simulink model "xieboduoji_13fangzhennow"  (R2023a)
settings: Solver=ode4  StartTime=0.0  StopTime=2.2  FixedStep=5e-7  RelTol=1e-3
undefined symbols (not defined in the file or in its folder): magnitude
libraries: simulink x417, spsRMSLib x70, spsCurrentMeasurementLib x32, spsVoltageMeasurementLib x31, powerlib_meascontrol x24, spsFourierLib x21, spsGroundLib x19, spsThreePhasePISectionLineLib x17, spsThreePhaseSeriesRLCBranchLib x14, spsdq0toAlphaBetaZeroLib x13, spsSeriesRLCBranchLib x11, spsUniversalBridgeLib x11
(part 11 of 12)

== system xieboduoji_13fangzhennow/node3/PV15kW3/谐波检测/Subsystem/Sub5 ==
  In1 : Inport
  Add : Sum
  Constant1 : Constant  Value=10*pi/180
  Constant{10,12,15,17} (4 alike) : Constant  Value=100*pi
  Constant11 : Constant  Value=19
  Constant2 : Constant  Value=10*pi/180
  Cos : Trigonometry  Operator=cos
  Cos1 : Trigonometry  Operator=cos
  Cos2 : Trigonometry
  Cos3 : Trigonometry
  Delay : Delay  DelayLength=400  SampleTime=5e-5
  Delay1 : Delay  DelayLength=1  SampleTime=5e-5
  Delay2 : Delay  DelayLength=1  SampleTime=5e-5
  Discrete PID Controller : slpidlib/PID Controller  Controller=P  Form=Parallel  TimeDomain=Discrete-time  UseExternalTs=off  SampleTime=5e-5  IntegratorMethod=Forward Euler  FilterMethod=Forward Euler  ControllerParametersSource=internal  P=1  I=1  UseKiTs=off  D=0  N=100  UseFilter=on  TunerSelectOption=Transfer Function Based (PID Tuner App)  InitialConditionSource=internal  InitialConditionForIntegrator=0  InitialConditionForFilter=0  DifferentiatorICPrevScaledInput=0  ExternalReset=none  TrackingMode=off  Kt=1  LimitOutput=off  SatLimitsSource=internal  UpperSaturationLimit=inf  LowerSaturationLimit=-inf  LinearizeAsGain=off  AntiWindupMode=none  Kb=1  LimitIntegrator=off  UpperIntegratorSaturationLimit=inf  LowerIntegratorSaturationLimit=-inf  POutMin=[]  POutMax=[]  IOutMin=[]  IOutMax=[]  DOutMin=[]  DOutMax=[]  NOutMin=[]  NOutMax=[]  SumOutMin=[]  SumOutMax=[]  SaturationOutMin=[]  SaturationOutMax=[]  PParamMin=[]  PParamMax=[]  IParamMin=[]  IParamMax=[]  DParamMin=[]  DParamMax=[]  NParamMin=[]  NParamMax=[]  KbParamMin=[]  KbParamMax=[]  KtParamMin=[]  KtParamMax=[]  KbOutMin=[]  KbOutMax=[]  KtOutMin=[]  KtOutMax=[]  IntegratorOutMin=[]  IntegratorOutMax=[]  FilterOutMin=[]  FilterOutMax=[]  SumI1OutMin=[]  SumI1OutMax=[]  SumI2OutMin=[]  SumI2OutMax=[]  SumI3OutMin=[]  SumI3OutMax=[]  SumI4OutMin=[]  SumI4OutMax=[]  SumDOutMin=[]  SumDOutMax=[]  DifferentiatorOutMin=[]  DifferentiatorOutMax=[]  FilterDiffOutCoefMin=[]  FilterDiffOutCoefMax=[]  ReciprocalOutMin=[]  ReciprocalOutMax=[]  SumDenOutMin=[]  SumDenOutMax=[]  SumNumOutMin=[]  SumNumOutMax=[]  DivideOutMin=[]  DivideOutMax=[]  UdiffTsProdOutMin=[]  UdiffTsProdOutMax=[]  NTsProdOutMin=[]  NTsProdOutMax=[]  UintegralTsProdOutMin=[]  UintegralTsProdOutMax=[]  UngainTsProdOutMin=[]  UngainTsProdOutMax=[]  ClampingZeroOutDataTypeStr=Inherit: Inherit via back propagation  ClampingZeroOutMin=[]  ClampingZeroOutMax=[]  FilterDenConstantOutDataTypeStr=Inherit: Inherit via back propagation  FilterDenConstantOutMin=[]  FilterDenConstantOutMax=[]  PCopyOutDataTypeStr=Inherit: Inherit via back propagation  PCopyOutMin=[]  PCopyOutMax=[]  NCopyOutDataTypeStr=Inherit: Inherit via back propagation  NCopyOutMin=[]  NCopyOutMax=[]  IntegratorContinuousStateAttributes=''  IntegratorStateMustResolveToSignalObject=off  IntegratorRTWStateStorageClass=Auto  FilterContinuousStateAttributes=''  FilterStateMustResolveToSignalObject=off  FilterRTWStateStorageClass=Auto  ParallelPVariant=InternalParameters  IdealPVariant=Disabled  IVariant=Disabled  DVariant=Disabled  IntegratorVariant=Disabled  SatVariant=Disabled  AWVariant=Disabled  PCopyVariant=Disabled  TRVariant=Disabled  FdbkBlocksVariant=Forward  IdealPFdbkVariant=Disabled  SatFdbkVariant=Disabled  DerivativeFilterVariant=Disabled  NVariant=Disabled  NCopyVariant=Disabled_SignalSpec  FilterICVariant=Disabled  IntegratorICVariant=Disabled  ExternalResetVariant=Disabled  TRSumVariant=Passthrough  SumFdbkVariant=Disabled  SumVariant=Passthrough_P  TsampFilterVariant=InternalTs  TsampNgainVariant=Passthrough  TsampIntegralVariant=Disabled_SignalSpec  ExternalSaturationOutDataTypeStr=Inherit: Same as second input
  Discrete PID Controller1 : slpidlib/PID Controller  Controller=P  Form=Parallel  TimeDomain=Discrete-time  UseExternalTs=off  SampleTime=5e-5  IntegratorMethod=Forward Euler  FilterMethod=Forward Euler  ControllerParametersSource=internal  P=1  I=1  UseKiTs=off  D=0  N=100  UseFilter=on  TunerSelectOption=Transfer Function Based (PID Tuner App)  InitialConditionSource=internal  InitialConditionForIntegrator=0  InitialConditionForFilter=0  DifferentiatorICPrevScaledInput=0  ExternalReset=none  TrackingMode=off  Kt=1  LimitOutput=off  SatLimitsSource=internal  UpperSaturationLimit=inf  LowerSaturationLimit=-inf  LinearizeAsGain=off  AntiWindupMode=none  Kb=1  LimitIntegrator=off  UpperIntegratorSaturationLimit=inf  LowerIntegratorSaturationLimit=-inf  POutMin=[]  POutMax=[]  IOutMin=[]  IOutMax=[]  DOutMin=[]  DOutMax=[]  NOutMin=[]  NOutMax=[]  SumOutMin=[]  SumOutMax=[]  SaturationOutMin=[]  SaturationOutMax=[]  PParamMin=[]  PParamMax=[]  IParamMin=[]  IParamMax=[]  DParamMin=[]  DParamMax=[]  NParamMin=[]  NParamMax=[]  KbParamMin=[]  KbParamMax=[]  KtParamMin=[]  KtParamMax=[]  KbOutMin=[]  KbOutMax=[]  KtOutMin=[]  KtOutMax=[]  IntegratorOutMin=[]  IntegratorOutMax=[]  FilterOutMin=[]  FilterOutMax=[]  SumI1OutMin=[]  SumI1OutMax=[]  SumI2OutMin=[]  SumI2OutMax=[]  SumI3OutMin=[]  SumI3OutMax=[]  SumI4OutMin=[]  SumI4OutMax=[]  SumDOutMin=[]  SumDOutMax=[]  DifferentiatorOutMin=[]  DifferentiatorOutMax=[]  FilterDiffOutCoefMin=[]  FilterDiffOutCoefMax=[]  ReciprocalOutMin=[]  ReciprocalOutMax=[]  SumDenOutMin=[]  SumDenOutMax=[]  SumNumOutMin=[]  SumNumOutMax=[]  DivideOutMin=[]  DivideOutMax=[]  UdiffTsProdOutMin=[]  UdiffTsProdOutMax=[]  NTsProdOutMin=[]  NTsProdOutMax=[]  UintegralTsProdOutMin=[]  UintegralTsProdOutMax=[]  UngainTsProdOutMin=[]  UngainTsProdOutMax=[]  ClampingZeroOutDataTypeStr=Inherit: Inherit via back propagation  ClampingZeroOutMin=[]  ClampingZeroOutMax=[]  FilterDenConstantOutDataTypeStr=Inherit: Inherit via back propagation  FilterDenConstantOutMin=[]  FilterDenConstantOutMax=[]  PCopyOutDataTypeStr=Inherit: Inherit via back propagation  PCopyOutMin=[]  PCopyOutMax=[]  NCopyOutDataTypeStr=Inherit: Inherit via back propagation  NCopyOutMin=[]  NCopyOutMax=[]  IntegratorContinuousStateAttributes=''  IntegratorStateMustResolveToSignalObject=off  IntegratorRTWStateStorageClass=Auto  FilterContinuousStateAttributes=''  FilterStateMustResolveToSignalObject=off  FilterRTWStateStorageClass=Auto  ParallelPVariant=InternalParameters  IdealPVariant=Disabled  IVariant=Disabled  DVariant=Disabled  IntegratorVariant=Disabled  SatVariant=Disabled  AWVariant=Disabled  PCopyVariant=Disabled  TRVariant=Disabled  FdbkBlocksVariant=Forward  IdealPFdbkVariant=Disabled  SatFdbkVariant=Disabled  DerivativeFilterVariant=Disabled  NVariant=Disabled  NCopyVariant=Disabled_SignalSpec  FilterICVariant=Disabled  IntegratorICVariant=Disabled  ExternalResetVariant=Disabled  TRSumVariant=Passthrough  SumFdbkVariant=Disabled  SumVariant=Passthrough_P  TsampFilterVariant=InternalTs  TsampNgainVariant=Passthrough  TsampIntegralVariant=Disabled_SignalSpec  ExternalSaturationOutDataTypeStr=Inherit: Same as second input
  Divide{,1..3} (4 alike) : Product  Inputs=***
  Dot Product{,1..5} (6 alike) : DotProduct  OutDataTypeStr=Inherit: Inherit via internal rule
  Gain : Gain  Gain=2/400
  Gain10 : Gain  Gain=2/400
  Ramp{,1..3} (4 alike) : simulink/Sources/Ramp  slope=1  start=0  InitialOutput=0
  Sqrt : Sqrt
  Sum{,1,3,9,18} (5 alike) : Sum  Inputs=|++
  Sum2 : Sum  Inputs=-+|
  u11 : Outport
  Out2 : Outport  Port=2
  wires:
  Constant17/1 -> Divide3/2
  Ramp/1 -> Divide/3
  Sum2/1 -> Dot Product2/1, Dot Product/2
  Divide/1 -> Cos/1
  Cos/1 -> Dot Product/1
  Dot Product/1 -> Gain/1
  Cos1/1 -> Dot Product1/1
  In1/1 -> Delay/1, Sum2/2
  Constant15/1 -> Divide2/2
  Sum18/1 -> Dot Product4/1, Discrete PID Controller1/1, Delay2/1
  [thk] -> Divide3/1
  [thk] -> Divide2/1
  Dot Product4/1 -> Sum9/2
  [thk] -> Divide1/1
  Ramp3/1 -> Divide3/3
  Delay1/1 -> Sum3/2
  Cos2/1 -> Dot Product2/2
  Dot Product2/1 -> Gain10/1
  Cos3/1 -> Dot Product4/2
  Divide2/1 -> Cos2/1
  Constant12/1 -> Divide1/2
  Ramp1/1 -> Divide1/3
  Delay/1 -> Sum2/1
  Sum3/1 -> Discrete PID Controller/1, Dot Product1/2, Delay1/1
  Gain10/1 -> Sum18/1
  Delay2/1 -> Sum18/2
  Constant10/1 -> Divide/2
  Ramp2/1 -> Divide2/3
  Gain/1 -> Sum3/1
  Dot Product1/1 -> Sum9/1
  Sum9/1 -> u11/1
  Constant11/1 -> [thk]
  [thk] -> Divide/1
  Dot Product3/1 -> Add/1
  Dot Product5/1 -> Add/2
  Add/1 -> Sqrt/1
  Sqrt/1 -> Out2/1
  Discrete PID Controller/1 -> Dot Product3/1, Dot Product3/2
  Discrete PID Controller1/1 -> Dot Product5/2, Dot Product5/1
  Divide1/1 -> Sum/1
  Sum/1 -> Cos1/1
  Divide3/1 -> Sum1/1
  Sum1/1 -> Cos3/1
  Constant1/1 -> Sum/2
  Constant2/1 -> Sum1/2

== system xieboduoji_13fangzhennow/node3/PV15kW3/谐波检测/Subsystem/Sub6 ==
  In1 : Inport
  Constant1 : Constant  Value=-60*pi/180
  Constant{10,12,15,17} (4 alike) : Constant  Value=100*pi
  Constant11 : Constant  Value=5
  Constant2 : Constant  Value=-60*pi/180
  Cos : Trigonometry  Operator=cos
  Cos1 : Trigonometry  Operator=cos
  Cos2 : Trigonometry
  Cos3 : Trigonometry
  Delay : Delay  DelayLength=400  SampleTime=5e-5
  Delay1 : Delay  DelayLength=1  SampleTime=5e-5
  Delay2 : Delay  DelayLength=1  SampleTime=5e-5
  Divide{,1..3} (4 alike) : Product  Inputs=***
  Dot Product{,1..2,4} (4 alike) : DotProduct  OutDataTypeStr=Inherit: Inherit via internal rule
  Gain : Gain  Gain=2/400
  Gain10 : Gain  Gain=2/400
  Ramp{,1..3} (4 alike) : simulink/Sources/Ramp  slope=1  start=0  InitialOutput=0
  Sum{,1,3,9,18} (5 alike) : Sum  Inputs=|++
  Sum2 : Sum  Inputs=-+|
  u1 : Outport
  wires:
  [thk] -> Divide/1
  Constant11/1 -> [thk]
  Sum9/1 -> u1/1
  Dot Product1/1 -> Sum9/1
  Gain/1 -> Sum3/1
  Ramp2/1 -> Divide2/3
  Constant10/1 -> Divide/2
  Delay2/1 -> Sum18/2
  Gain10/1 -> Sum18/1
  Sum3/1 -> Delay1/1, Dot Product1/2
  Delay/1 -> Sum2/1
  Ramp1/1 -> Divide1/3
  Constant12/1 -> Divide1/2
  Divide2/1 -> Cos2/1
  Cos3/1 -> Dot Product4/2
  Dot Product2/1 -> Gain10/1
  Cos2/1 -> Dot Product2/2
  Delay1/1 -> Sum3/2
  Ramp3/1 -> Divide3/3
  [thk] -> Divide1/1
  Dot Product4/1 -> Sum9/2
  [thk] -> Divide2/1
  [thk] -> Divide3/1
  Sum18/1 -> Delay2/1, Dot Product4/1
  Constant15/1 -> Divide2/2
  In1/1 -> Sum2/2, Delay/1
  Dot Product/1 -> Gain/1
  Cos/1 -> Dot Product/1
  Divide/1 -> Cos/1
  Sum2/1 -> Dot Product/2, Dot Product2/1
  Ramp/1 -> Divide/3
  Constant17/1 -> Divide3/2
  Cos1/1 -> Dot Product1/1
  Divide1/1 -> Sum/1
  Sum/1 -> Cos1/1
  Sum1/1 -> Cos3/1
  Divide3/1 -> Sum1/1

== system xieboduoji_13fangzhennow/node3/PV15kW3/谐波检测/Subsystem/Sub7 ==
  In1 : Inport
  Constant1 : Constant  Value=-60*pi/180
  Constant{10,12,15,17} (4 alike) : Constant  Value=100*pi
  Constant11 : Constant  Value=7
  Constant2 : Constant  Value=-60*pi/180
  Cos : Trigonometry  Operator=cos
  Cos1 : Trigonometry  Operator=cos
  Cos2 : Trigonometry
  Cos3 : Trigonometry
  Delay : Delay  DelayLength=400  SampleTime=5e-5
  Delay1 : Delay  DelayLength=1  SampleTime=5e-5
  Delay2 : Delay  DelayLength=1  SampleTime=5e-5
  Divide{,1..3} (4 alike) : Product  Inputs=***
  Dot Product{,1..2,4} (4 alike) : DotProduct  OutDataTypeStr=Inherit: Inherit via internal rule
  Gain : Gain  Gain=2/400
  Gain10 : Gain  Gain=2/400
  Ramp{,1..3} (4 alike) : simulink/Sources/Ramp  slope=1  start=0  InitialOutput=0
  Sum{,1,3,9,18} (5 alike) : Sum  Inputs=|++
  Sum2 : Sum  Inputs=-+|
  u1 : Outport
  wires:
  Divide3/1 -> Sum1/1
  Sum1/1 -> Cos3/1
  Sum/1 -> Cos1/1
  Divide1/1 -> Sum/1
  Cos1/1 -> Dot Product1/1
  Constant17/1 -> Divide3/2
  Ramp/1 -> Divide/3
  Sum2/1 -> Dot Product2/1, Dot Product/2
  Divide/1 -> Cos/1
  Cos/1 -> Dot Product/1
  Dot Product/1 -> Gain/1
  In1/1 -> Delay/1, Sum2/2
  Constant15/1 -> Divide2/2
  Sum18/1 -> Dot Product4/1, Delay2/1
  [thk] -> Divide3/1
  [thk] -> Divide2/1
  Dot Product4/1 -> Sum9/2
  [thk] -> Divide1/1
  Ramp3/1 -> Divide3/3
  Delay1/1 -> Sum3/2
  Cos2/1 -> Dot Product2/2
  Dot Product2/1 -> Gain10/1
  Cos3/1 -> Dot Product4/2
  Divide2/1 -> Cos2/1
  Constant12/1 -> Divide1/2
  Ramp1/1 -> Divide1/3
  Delay/1 -> Sum2/1
  Sum3/1 -> Dot Product1/2, Delay1/1
  Gain10/1 -> Sum18/1
  Delay2/1 -> Sum18/2
  Constant10/1 -> Divide/2
  Ramp2/1 -> Divide2/3
  Gain/1 -> Sum3/1
  Dot Product1/1 -> Sum9/1
  Sum9/1 -> u1/1
  Constant11/1 -> [thk]
  [thk] -> Divide/1

== system xieboduoji_13fangzhennow/node3/PV15kW3/谐波检测/Subsystem/Sub8 ==
  In1 : Inport
  Constant1 : Constant  Value=-15*pi/180
  Constant{10,12,15,17} (4 alike) : Constant  Value=100*pi
  Constant11 : Constant  Value=11
  Constant2 : Constant  Value=-15*pi/180
  Cos : Trigonometry  Operator=cos
  Cos2 : Trigonometry
  Cos3 : Trigonometry
  Cos4 : Trigonometry  Operator=cos
  Delay : Delay  DelayLength=400  SampleTime=5e-5
  Delay1 : Delay  DelayLength=1  SampleTime=5e-5
  Delay2 : Delay  DelayLength=1  SampleTime=5e-5
  Divide{,1..3} (4 alike) : Product  Inputs=***
  Dot Product{,1..2,4} (4 alike) : DotProduct  OutDataTypeStr=Inherit: Inherit via internal rule
  Gain : Gain  Gain=2/400
  Gain10 : Gain  Gain=2/400
  Ramp{,1..3} (4 alike) : simulink/Sources/Ramp  slope=1  start=0  InitialOutput=0
  Sum{,1,3,9,18} (5 alike) : Sum  Inputs=|++
  Sum2 : Sum  Inputs=-+|
  u5 : Outport
  wires:
  Sum1/1 -> Cos3/1
  Constant1/1 -> Sum1/2
  Divide3/1 -> Sum1/1
  Cos4/1 -> Dot Product1/1
  Sum/1 -> Cos4/1
  Constant2/1 -> Sum/2
  Divide1/1 -> Sum/1
  Constant17/1 -> Divide3/2
  Ramp/1 -> Divide/3
  Sum2/1 -> Dot Product2/1, Dot Product/2
  Divide/1 -> Cos/1
  Cos/1 -> Dot Product/1
  Dot Product/1 -> Gain/1
  In1/1 -> Delay/1, Sum2/2
  Constant15/1 -> Divide2/2
  Sum18/1 -> Dot Product4/1, Delay2/1
  [thk] -> Divide3/1
  [thk] -> Divide2/1
  Dot Product4/1 -> Sum9/2
  [thk] -> Divide1/1
  Ramp3/1 -> Divide3/3
  Delay1/1 -> Sum3/2
  Cos2/1 -> Dot Product2/2
  Dot Product2/1 -> Gain10/1
  Cos3/1 -> Dot Product4/2
  Divide2/1 -> Cos2/1
  Constant12/1 -> Divide1/2
  Ramp1/1 -> Divide1/3
  Delay/1 -> Sum2/1
  Sum3/1 -> Dot Product1/2, Delay1/1
  Gain10/1 -> Sum18/1
  Delay2/1 -> Sum18/2
  Constant10/1 -> Divide/2
  Ramp2/1 -> Divide2/3
  Gain/1 -> Sum3/1
  Dot Product1/1 -> Sum9/1
  Sum9/1 -> u5/1
  Constant11/1 -> [thk]
  [thk] -> Divide/1

== system xieboduoji_13fangzhennow/node3/PV15kW3/谐波检测/Subsystem/Sub9 ==
  In1 : Inport
  Constant1 : Constant  Value=-15*pi/180
  Constant{10,12,15,17} (4 alike) : Constant  Value=100*pi
  Constant11 : Constant  Value=13
  Constant2 : Constant  Value=-15*pi/180
  Cos : Trigonometry  Operator=cos
  Cos1 : Trigonometry  Operator=cos
  Cos2 : Trigonometry
  Cos3 : Trigonometry
  Delay : Delay  DelayLength=400  SampleTime=5e-5
  Delay1 : Delay  DelayLength=1  SampleTime=5e-5
  Delay2 : Delay  DelayLength=1  SampleTime=5e-5
  Divide{,1..3} (4 alike) : Product  Inputs=***
  Dot Product{,1..2,4} (4 alike) : DotProduct  OutDataTypeStr=Inherit: Inherit via internal rule
  Gain : Gain  Gain=2/400
  Gain10 : Gain  Gain=2/400
  Ramp{,1..3} (4 alike) : simulink/Sources/Ramp  slope=1  start=0  InitialOutput=0
  Sum{,1,3,9,18} (5 alike) : Sum  Inputs=|++
  Sum2 : Sum  Inputs=-+|
  u7 : Outport
  wires:
  Sum1/1 -> Cos3/1
  Constant1/1 -> Sum1/2
  Divide3/1 -> Sum1/1
  Sum/1 -> Cos1/1
  Constant2/1 -> Sum/2
  Divide1/1 -> Sum/1
  [thk] -> Divide/1
  Constant11/1 -> [thk]
  Sum9/1 -> u7/1
  Dot Product1/1 -> Sum9/1
  Gain/1 -> Sum3/1
  Ramp2/1 -> Divide2/3
  Constant10/1 -> Divide/2
  Delay2/1 -> Sum18/2
  Gain10/1 -> Sum18/1
  Sum3/1 -> Delay1/1, Dot Product1/2
  Delay/1 -> Sum2/1
  Ramp1/1 -> Divide1/3
  Constant12/1 -> Divide1/2
  Divide2/1 -> Cos2/1
  Cos3/1 -> Dot Product4/2
  Dot Product2/1 -> Gain10/1
  Cos2/1 -> Dot Product2/2
  Delay1/1 -> Sum3/2
  Ramp3/1 -> Divide3/3
  [thk] -> Divide1/1
  Dot Product4/1 -> Sum9/2
  [thk] -> Divide2/1
  [thk] -> Divide3/1
  Sum18/1 -> Delay2/1, Dot Product4/1
  Constant15/1 -> Divide2/2
  In1/1 -> Sum2/2, Delay/1
  Cos1/1 -> Dot Product1/1
  Dot Product/1 -> Gain/1
  Cos/1 -> Dot Product/1
  Divide/1 -> Cos/1
  Sum2/1 -> Dot Product/2, Dot Product2/1
  Ramp/1 -> Divide/3
  Constant17/1 -> Divide3/2

== system xieboduoji_13fangzhennow/node3/PV15kW3/谐波检测/Subsystem/Subsystem2 ==
  u1 : Inport
  u2 : Inport  Port=2
  u3 : Inport  Port=3
  u4 : Inport  Port=4
  u5 : Inport  Port=5
  u6 : Inport  Port=6
  u7 : Inport  Port=7
  u8 : Inport  Port=8
  u9 : Inport  Port=9
  u10 : Inport  Port=10
  u11 : Inport  Port=11
  u12 : Inport  Port=12
  Pul : DiscretePulseGenerator  PulseType=Time based  Period=5e-5  PulseWidth=40
  RMS1 : Subsystem  TreatAsAtomicUnit=on
  k1 : Outport  VectorParamsAs1DForOutWhenUnconnected=off
  k2 : Outport  Port=2  VectorParamsAs1DForOutWhenUnconnected=off
  k3 : Outport  Port=3  VectorParamsAs1DForOutWhenUnconnected=off
  k4 : Outport  Port=4  VectorParamsAs1DForOutWhenUnconnected=off
  k5 : Outport  Port=5  VectorParamsAs1DForOutWhenUnconnected=off
  k6 : Outport  Port=6  VectorParamsAs1DForOutWhenUnconnected=off
  wires:
  Pul/1 -> RMS1/Trigger
  u1/1 -> RMS1/1(u1)
  u2/1 -> RMS1/2(i1)
  u3/1 -> RMS1/3(u3)
  u4/1 -> RMS1/4(u4)
  u5/1 -> RMS1/5(u5)
  u6/1 -> RMS1/6(u6)
  RMS1/2(k2) -> k2/1
  RMS1/3(k3) -> k3/1
  RMS1/4(k4) -> k4/1
  RMS1/1(k1) -> k1/1
  RMS1/6(k6) -> k6/1
  RMS1/5(k5) -> k5/1
  u12/1 -> RMS1/12(u10)
  u11/1 -> RMS1/11(u9)
  u10/1 -> RMS1/10(u8)
  u9/1 -> RMS1/9(u7)
  u8/1 -> RMS1/8(i2)
  u7/1 -> RMS1/7(u2)

== system xieboduoji_13fangzhennow/node3/PV15kW3/谐波检测/Subsystem2/RMS1 ==
  u1 : Inport
  i1 : Inport  Port=2
  u3 : Inport  Port=3
  u4 : Inport  Port=4
  u5 : Inport  Port=5
  u6 : Inport  Port=6
  u2 : Inport  Port=7
  i2 : Inport  Port=8
  u7 : Inport  Port=9
  u8 : Inport  Port=10
  u9 : Inport  Port=11
  u10 : Inport  Port=12
  Trigger : TriggerPort  VariantControl=(inherit)
  Scope : Scope
  xiebodianliu : MATLAB Function  Commented=on  TreatAsAtomicUnit=on
  xunidiandao : MATLAB Function  TreatAsAtomicUnit=on
  k1 : Outport  VectorParamsAs1DForOutWhenUnconnected=off
  k2 : Outport  Port=2  VectorParamsAs1DForOutWhenUnconnected=off
  k3 : Outport  Port=3  VectorParamsAs1DForOutWhenUnconnected=off
  k4 : Outport  Port=4  VectorParamsAs1DForOutWhenUnconnected=off
  k5 : Outport  Port=5  VectorParamsAs1DForOutWhenUnconnected=off
  k6 : Outport  Port=6  VectorParamsAs1DForOutWhenUnconnected=off
  wires:
  xunidiandao/1(k1) -> k1/1
  u1/1 -> xunidiandao/1(u1)
  xunidiandao/2(k2) -> k2/1
  xunidiandao/3(k3) -> k3/1
  xunidiandao/4(k4) -> k4/1
  xunidiandao/5(k5) -> k5/1
  xunidiandao/6(k6) -> k6/1
  i1/1 -> xunidiandao/2(i1)
  u3/1 -> xunidiandao/3(u2)
  u4/1 -> xunidiandao/4(i2)
  u5/1 -> xunidiandao/5(u3)
  u6/1 -> xunidiandao/6(i3)
  u10/1 -> xunidiandao/12(i6)
  u9/1 -> xunidiandao/11(u6)
  u8/1 -> xunidiandao/10(i5)
  u7/1 -> xunidiandao/9(u5)
  i2/1 -> xunidiandao/8(i4)
  u2/1 -> xunidiandao/7(u4)
  xunidiandao/7(k0) -> Scope/1

== system xieboduoji_13fangzhennow/node12/PV15kW3/谐波检测/Subsystem/Subsystem2/RMS1 ==
  u1 : Inport
  i1 : Inport  Port=2
  u3 : Inport  Port=3
  u4 : Inport  Port=4
  u5 : Inport  Port=5
  u6 : Inport  Port=6
  u2 : Inport  Port=7
  i2 : Inport  Port=8
  u7 : Inport  Port=9
  u8 : Inport  Port=10
  u9 : Inport  Port=11
  u10 : Inport  Port=12
  Trigger : TriggerPort  VariantControl=(inherit)
  Scope : Scope
  xiebodianliu : MATLAB Function  TreatAsAtomicUnit=on
  k1 : Outport  VectorParamsAs1DForOutWhenUnconnected=off
  k2 : Outport  Port=2  VectorParamsAs1DForOutWhenUnconnected=off
  k3 : Outport  Port=3  VectorParamsAs1DForOutWhenUnconnected=off
  k4 : Outport  Port=4  VectorParamsAs1DForOutWhenUnconnected=off
  k5 : Outport  Port=5  VectorParamsAs1DForOutWhenUnconnected=off
  k6 : Outport  Port=6  VectorParamsAs1DForOutWhenUnconnected=off
  wires:
  xiebodianliu/1(k1) -> k1/1
  u1/1 -> xiebodianliu/1(u1)
  xiebodianliu/2(k2) -> k2/1
  xiebodianliu/3(k3) -> k3/1
  xiebodianliu/4(k4) -> k4/1
  xiebodianliu/5(k5) -> k5/1
  xiebodianliu/6(k6) -> k6/1
  i1/1 -> xiebodianliu/2(i1)
  u3/1 -> xiebodianliu/3(u2)
  u4/1 -> xiebodianliu/4(i2)
  u5/1 -> xiebodianliu/5(u3)
  u6/1 -> xiebodianliu/6(i3)
  u10/1 -> xiebodianliu/12(i6)
  u9/1 -> xiebodianliu/11(u6)
  u8/1 -> xiebodianliu/10(i5)
  u7/1 -> xiebodianliu/9(u5)
  i2/1 -> xiebodianliu/8(i4)
  u2/1 -> xiebodianliu/7(u4)
  xiebodianliu/7(k0) -> Scope/1

== system xieboduoji_13fangzhennow/node3/PV15kW2/谐波检测/DFT6-24A1/Subsystem9/integral  ==
  di : Inport
  Trigger : TriggerPort  VariantControl=(inherit)
  Embedded MATLAB Function : MATLAB Function  TreatAsAtomicUnit=on
  w : Outport
  wires:
  Embedded MATLAB Function/1(w) -> w/1
  di/1 -> Embedded MATLAB Function/1(er)

== system xieboduoji_13fangzhennow/node3/PV15kW3/谐波检测/Subsystem/Subsystem2/RMS1 ==
  u1 : Inport
  i1 : Inport  Port=2
  u3 : Inport  Port=3
  u4 : Inport  Port=4
  u5 : Inport  Port=5
  u6 : Inport  Port=6
  u2 : Inport  Port=7
  i2 : Inport  Port=8
  u7 : Inport  Port=9
  u8 : Inport  Port=10
  u9 : Inport  Port=11
  u10 : Inport  Port=12
  Trigger : TriggerPort  VariantControl=(inherit)
  Scope : Scope
  xiebodianliu : MATLAB Function  TreatAsAtomicUnit=on
  xiebodianliu1 : MATLAB Function  Commented=on  TreatAsAtomicUnit=on
  k1 : Outport  VectorParamsAs1DForOutWhenUnconnected=off
  k2 : Outport  Port=2  VectorParamsAs1DForOutWhenUnconnected=off
  k3 : Outport  Port=3  VectorParamsAs1DForOutWhenUnconnected=off
  k4 : Outport  Port=4  VectorParamsAs1DForOutWhenUnconnected=off
  k5 : Outport  Port=5  VectorParamsAs1DForOutWhenUnconnected=off
  k6 : Outport  Port=6  VectorParamsAs1DForOutWhenUnconnected=off
  wires:
  xiebodianliu/1(k1) -> k1/1
  u1/1 -> xiebodianliu/1(u1)
  xiebodianliu/2(k2) -> k2/1
  xiebodianliu/3(k3) -> k3/1
  xiebodianliu/4(k4) -> k4/1
  xiebodianliu/5(k5) -> k5/1
  xiebodianliu/6(k6) -> k6/1
  i1/1 -> xiebodianliu/2(i1)
  u3/1 -> xiebodianliu/3(u2)
  u4/1 -> xiebodianliu/4(i2)
  u5/1 -> xiebodianliu/5(u3)
  u6/1 -> xiebodianliu/6(i3)
  u10/1 -> xiebodianliu/12(i6)
  u9/1 -> xiebodianliu/11(u6)
  u8/1 -> xiebodianliu/10(i5)
  u7/1 -> xiebodianliu/9(u5)
  i2/1 -> xiebodianliu/8(i4)
  u2/1 -> xiebodianliu/7(u4)
  xiebodianliu/7(k0) -> Scope/1

== matlab function xieboduoji_13fangzhennow/node3/Subsystem2/RMS1/xunidiandao ==
  data: y1 output; u1 input; u2 input; u3 input; u4 input; u5 input; u6 input; y11 output; y2 output; y22 output; y3 output; y33 output; y4 output; y44 output; y5 output; y55 output; y6 output; y66 output; x output
function [y1,y11,y2,y22,y3,y33,y4,y44,y5,y55,y6,y66,x] = Algorithm(u1,u2,u3,u4,u5,u6)

%控制器参数
T=5e-5;
persistent time;
persistent sum1 sum2 sum3 sum4 sum5 sum6;
persistent sum11 sum22 sum33 sum44 sum55 sum66;
persistent a1 a11 a2 a22 a3 a33 a4 a44 a5 a55 a6 a66
dataType = 'double';

%首次赋值
 if isempty(time)
time=20e-5;
sum1=0;sum2=0;sum3=0;sum4=0;sum5=0;sum6=0;
sum11=0;sum22=0;sum33=0;sum44=0;sum55=0;sum66=0;
a1=0;a11=0;a2=0;a22=0;a3=0;a33=0;a4=0;a44=0;a5=0;a55=0;a6=0;a66=0;
 end

 time=time+T;
  
 if (time>=0.9)&&(time<1.0)
     sum1=sum1+u1;sum2=sum2+u2;sum3=sum3+u3;
     sum4=sum4+u4;sum5=sum5+u5;sum6=sum6+u6;
 end
 if time>=1.0
     a1=sum1*0.0005;a2=sum2*0.0005;a3=sum3*0.0005;
     a4=sum4*0.0005;a5=sum5*0.0005;a6=sum6*0.0005;
 end
  if (time>=1.9)&&(time<2.0)
     sum11=sum11+u1;sum22=sum22+u2;sum33=sum33+u3;
     sum44=sum44+u4;sum55=sum55+u5;sum66=sum66+u6;
 end
 if time>=2.0
     a11=sum11*0.0005;a22=sum22*0.0005;a33=sum33*0.0005;
     a44=sum44*0.0005;a55=sum55*0.0005;a66=sum66*0.0005;
 end
 y1=a1;y2=a2;y3=a3;y4=a4;y5=a5;y6=a6;
 y11=a11;y22=a22;y33=a33;y44=a44;y55=a55;y66=a66;x=time+sum1;
end

== matlab function xieboduoji_13fangzhennow/node14/PV15kW3/谐波检测/Subsystem2/RMS1/xunidiandao ==
  data: k1 output; u1 input; i1 input; u2 input; i2 input; u3 input; i3 input; u4 input; i4 input; u5 input; i5 input; u6 input; k2 output; k3 output; k4 output; k5 output; k6 output; i6 input; k0 output
function [k1,k2,k3,k4,k5,k6,k0] = Algorithm(u1,i1,u2,i2,u3,i3,u4,i4,u5,i5,u6,i6)

%控制器参数
T=5e-5;
kp=0.01;
persistent low lim im k time;
persistent k11 k22 k33 k44 k55 k66 sumc;
persistent h1 flg1 sum1 out1 bao1 ki1;
persistent h2 flg2 sum2 out2 bao2 ki2;
persistent h3 flg3 sum3 out3 bao3 ki3;
persistent h4 flg4 sum4 out4 bao4 ki4;
persistent h5 flg5 sum5 out5 bao5 ki5;
persistent h6 flg6 sum6 out6 bao6 ki6;
dataType = 'double';

%首次赋值
 if isempty(k)
 low=311*0.25;lim=5;im=0;k=1;time=5e-5;%1.1
 k11=0;k22=0;k33=0;k44=0;k55=0;k66=0;sumc=0;
 h1=1;flg1=1;sum1=1;out1=1;bao1=0;ki1=25;
 h2=1;flg2=1;sum2=1;out2=1;bao2=0;ki2=25;
 h3=1;flg3=1;sum3=1;out3=1;bao3=0;ki3=25;
 h4=1;flg4=1;sum4=1;out4=1;bao4=0;ki4=25;
 h5=1;flg5=1;sum5=1;out5=1;bao5=0;ki5=25;
 h6=1;flg6=1;sum6=1;out6=1;bao6=0;ki6=25;
 end
   if (flg5==0)&&(flg6==0)
       sumc=sqrt((i5*out5)^2+(i6*out6)^2);
    if sumc>lim
        k11=k11*lim/sumc;out1=k11;sum1=k11;
        k22=k22*lim/sumc;out2=k22;sum2=k22;
        k33=k33*lim/sumc;out3=k33;sum3=k33;
        k44=k44*lim/sumc;out4=k44;sum4=k44;
        k55=k55*lim/sumc;out5=k55;sum5=k55;
        k66=k66*lim/sumc;out6=k66;sum6=k66;end 
   end
    if flg1==1
      h1=1;
    else h1=out1/k;end
    if flg2==1
      h2=1;
    else h2=out2/k;end
    if flg3==1
      h3=1;
    else h3=out3/k;end   
    if flg4==1
      h4=1;
    else h4=out4/k;end   
    if flg5==1
      h5=1;
    else h5=out5/k;end 
    if flg6==1
      h6=1;
    else h6=out6/k;end   
 im=sqrt((i1*h1)^2+(i2*h2)^2+(i3*h3)^2+(i4*h4)^2+(i5*h5)^2+(i6*h6)^2);%
 time=time+T;  
 k=lim/im;
     if k>3
     k=3;end
     if flg1==1
     k11=k;end
     if flg2==1
     k22=k;end 
     if flg3==1
     k33=k;end
     if flg4==1
     k44=k;end
     if flg5==1
     k55=k;end
     if flg6==1
     k66=k;end
  
 if time<1
     k11=0;k22=0;k33=0;k44=0;k55=0;k66=0;
 end
 if time>=1
     % if time>=1.4
     % low=1.02;end%1.02
     % if time>=1.7
     % low=0.512;end%0.512
  if time>=1.4
lim=10.6-time*4.0;lim1=10.6-time*4.0;
    if lim<4
    lim=4;lim1=4;
    end
  end
  
 er6=u6*1.414-low;er5=u5*1.414-low;
    if (er5<-0.06)||(er5>0.06)
         if (er5>0.06)%
         flg5=1;end
         if (er5<-0.06) 
          if flg5==1
          sum5=k;out5=k;end
         flg5=0;end   
    sum5=ki5*T*er5+sum5;out5=kp*er5+sum5;
        if flg5==0 
        k55=out5;end
     if(out5>k)
     flg5=1;out5=k;ki5=0;bao5=1;end
     if(out5<0)
     out5=0;ki5=0;bao5=1;end
     if(bao5==0)
     ki5=40;end
     bao5=0;
   end
    if (er6<-0.06)||(er6>0.06)
         if (er6>0.06)%
         flg6=1;end
         if (er6<-0.06) 
           if flg6==1
           sum6=k;out6=k;end
         flg6=0;end   
     sum6=ki6*T*er6+sum6; out6=kp*er6+sum6;
        if flg6==0 
        k66=out6;end
     if(out6>k)
     flg6=1;out6=k;ki6=0;bao6=1;end
     if(out6<0)
     out6=0;ki6=0;bao6=1;end
     if(bao6==0)
     ki6=40;end
     bao6=0;
    end
 end
 
 k1=k11;k2=k22;k3=k33;k4=k44;k5=k55;k6=k66;k0=flg6;
end

== matlab function xieboduoji_13fangzhennow/node12/PV15kW3/Subsystem9/integral /Embedded MATLAB Function ==
  data: er input; w output
function w  = Algorithm(er)

%控制器参数
Ts=10e-5;%控制周期，原始0.3-6
Kp=0.3;Ki0=8;n=35;
persistent n_sum dcbaohe Ki;
dataType = 'double';

%首次赋值
if isempty(n_sum)
    n_sum=0;dcbaohe=0;Ki=Ki0;
end
 
     n_sum=Ki*Ts*(er)+n_sum;
     outn=Kp*(er)+n_sum;
     if(outn>n)
     outn=n;Ki=0;dcbaohe=1;
     end
     if(outn<-n)
     outn=-n;Ki=0;dcbaohe=1;
     end
     if(dcbaohe==0)
         Ki=Ki0;
     end
     dcbaohe=0;
     
  w=outn; 
end

== matlab function xieboduoji_13fangzhennow/node12/PV15kW3/改进PLL1/PI/Embedded MATLAB Function ==
  data: Vgq input; w output
function w  = Algorithm(Vgq)

%控制器参数
T=5e-5;%控制周期

Kpllp=0.2;
Kplli=4;

persistent PLLsum;
persistent nsum2;

dataType = 'double';

%首次赋值
if isempty(PLLsum)
    PLLsum=0;
    nsum2=0;
end


w=Kpllp*Vgq+Kplli*(T*Vgq+PLLsum);
PLLsum=T*Vgq+PLLsum;
end

== matlab function xieboduoji_13fangzhennow/node3/PV15kW3/谐波检测/Subsystem/Subsystem2/RMS1/xiebodianliu ==
  data: k1 output; u1 input; i1 input; u2 input; i2 input; u3 input; i3 input; u4 input; i4 input; u5 input; i5 input; u6 input; k2 output; k3 output; k4 output; k5 output; k6 output; i6 input; k0 output
function [k1,k2,k3,k4,k5,k6,k0] = Algorithm(u1,i1,u2,i2,u3,i3,u4,i4,u5,i5,u6,i6)

%控制器参数
T=5e-5;
kp=0.01;
persistent lim lim1 im k time;
persistent k11 k22 k33 k44 k55 k66;
persistent flg1 flg2 flg3 flg4 flg5 flg6;
dataType = 'double';

%首次赋值
 if isempty(k)
 lim=5;lim1=5;im=0;k=1;time=5e-5;
 k11=0;k22=0;k33=0;k44=0;k55=0;k66=0;
 flg1=1; flg2=1; flg3=1; flg4=1; flg5=1; flg6=1;
 end
h1=1/0.6464;h2=1/0.7219;h3=1/1;
h4=1/0.9880;h5=1/0.5562;h6=1/0.6416;

im=sqrt(flg1*i1^2+flg2*i2^2+flg3*i3^2+flg4*i4^2+flg5*i5^2+flg6*i6^2);
it=(lim^2-((1-flg1)*h1*i1)^2-((1-flg2)*h2*i2)^2-((1-flg3)*h3*i3)^2-((1-flg4)*h4*i4)^2-((1-flg5)*h5*i5)^2-((1-flg6)*h6*i6)^2);
 if it>=0
 lim1=sqrt(it);
  if im>0
  k=lim1/im;end
 else
 lim1=0;k=0.7;
 end
time=time+T;
 if k>2
 k=2;end
     if k>h1
      k11=h1;flg1=0;
      else
      flg1=1;k11=k;end
     if k>h2
      k22=h2;flg2=0;
      else
      flg2=1;k22=k;end
     if k>h3
      k33=h3;flg3=0;
      else
      flg3=1;k33=k;end
     if k>h4
      k44=h4;flg4=0;
      else
      flg4=1;k44=k;end
     if k>h5
      k55=h5;flg5=0;
      else
      flg5=1;k55=k;end
     if k>h6
      k66=h6;flg6=0;
      else
      flg6=1;k66=k;end

  
 if time<1
     k11=0;k22=0;k33=0;k44=0;k55=0;k66=0;
 end
 if time>=1.4
lim=10.6-time*4.0;lim1=10.6-time*4.0;
    if lim<4
    lim=4;lim1=4;
    end
 end
 
 k1=k11;k2=k22;k3=k33;k4=k44;k5=k55;k6=k66;k0=it;
end

== matlab function xieboduoji_13fangzhennow/node12/PV15kW3/谐波检测/Subsystem/Subsystem2/RMS1/xiebodianliu ==
  data: k1 output; u1 input; i1 input; u2 input; i2 input; u3 input; i3 input; u4 input; i4 input; u5 input; i5 input; u6 input; k2 output; k3 output; k4 output; k5 output; k6 output; i6 input; k0 output
function [k1,k2,k3,k4,k5,k6,k0] = Algorithm(u1,i1,u2,i2,u3,i3,u4,i4,u5,i5,u6,i6)

%控制器参数
T=5e-5;
kp=0.01;
persistent lim lim1 im k time;
persistent k11 k22 k33 k44 k55 k66;
persistent flg1 flg2 flg3 flg4 flg5 flg6;
dataType = 'double';

%首次赋值
 if isempty(k)
 lim=5;lim1=5;im=0;k=1;time=5e-5;
 k11=0;k22=0;k33=0;k44=0;k55=0;k66=0;
 flg1=1; flg2=1; flg3=1; flg4=1; flg5=1; flg6=1;
 end
h1=1/0.7237;h2=1/0.8217;h3=1/1;
h4=1/1;h5=1/1;h6=1/1;

im=sqrt(flg1*i1^2+flg2*i2^2+flg3*i3^2+flg4*i4^2+flg5*i5^2+flg6*i6^2);
it=(lim^2-((1-flg1)*h1*i1)^2-((1-flg2)*h2*i2)^2-((1-flg3)*h3*i3)^2-((1-flg4)*h4*i4)^2-((1-flg5)*h5*i5)^2-((1-flg6)*h6*i6)^2);
 if it>=0
 lim1=sqrt(it);
  if im>0
  k=lim1/im;end
 else
 lim1=0;k=0.7;
 end
time=time+T;
 if k>2
 k=2;end
     if k>h1
      k11=h1;flg1=0;
      else
      flg1=1;k11=k;end
     if k>h2
      k22=h2;flg2=0;
      else
      flg2=1;k22=k;end
     if k>h3
      k33=h3;flg3=0;
      else
      flg3=1;k33=k;end
     if k>h4
      k44=h4;flg4=0;
      else
      flg4=1;k44=k;end
     if k>h5
      k55=h5;flg5=0;
      else
      flg5=1;k55=k;end
     if k>h6
      k66=h6;flg6=0;
      else
      flg6=1;k66=k;end

  
 if time<1
     k11=0;k22=0;k33=0;k44=0;k55=0;k66=0;
 end
 if time>=1.4
lim=10.6-time*4.0;lim1=10.6-time*4.0;
    if lim<4
    lim=4;lim1=4;
    end
 end
 
 k1=k11;k2=k22;k3=k33;k4=k44;k5=k55;k6=k66;k0=it;
end

== matlab function xieboduoji_13fangzhennow/node3/PV15kW3/Subsystem9/integral /Embedded MATLAB Function ==
  data: er input; w output
function w  = Algorithm(er)

%控制器参数
Ts=10e-5;%控制周期，原始0.3-6
Kp=0.3;Ki0=8;n=35;
persistent n_sum dcbaohe Ki;
dataType = 'double';

%首次赋值
if isempty(n_sum)
    n_sum=0;dcbaohe=0;Ki=Ki0;
end
 
     n_sum=Ki*Ts*(er)+n_sum;
     outn=Kp*(er)+n_sum;
     if(outn>n)
     outn=n;Ki=0;dcbaohe=1;
     end
     if(outn<-n)
     outn=-n;Ki=0;dcbaohe=1;
     end
     if(dcbaohe==0)
         Ki=Ki0;
     end
     dcbaohe=0;
     
  w=outn; 
end

== matlab function xieboduoji_13fangzhennow/node12/PV15kW3/谐波检测/Subsystem2/RMS1/xunidiandao ==
  data: k1 output; u1 input; i1 input; u2 input; i2 input; u3 input; i3 input; u4 input; i4 input; u5 input; i5 input; u6 input; k2 output; k3 output; k4 output; k5 output; k6 output; i6 input; k0 output
function [k1,k2,k3,k4,k5,k6,k0] = Algorithm(u1,i1,u2,i2,u3,i3,u4,i4,u5,i5,u6,i6)

%控制器参数
T=5e-5;
kp=0.01;
persistent low lim im k time;
persistent k11 k22 k33 k44 k55 k66;
persistent h6 flg6 sum6 out6 bao6 ki6;
persistent h5 flg5 sum5 out5 bao5 ki5;
dataType = 'double';

%首次赋值
 if isempty(k)
 low=1.244;lim=5;im=0;k=1;time=5e-5;%1.1
 k11=0;k22=0;k33=0;k44=0;k55=0;k66=0;
 h6=1;flg6=1;sum6=1;out6=1;bao6=0;ki6=25;
 h5=1;flg5=1;sum5=1;out5=1;bao5=0;ki5=25;
 end
%    if (flg5==0)&&(flg6==0)
%     if sqrt((i5*out5)^2+(i6*out6)^2)>lim
%          if (flg5>flg6)
%              flg5=1;
%          else
%              flg6=1;
%          end
%     end
%    end  
    if flg5==1
      h5=1;
    else h5=out5/k;end 
    if flg6==1
      h6=1;
    else h6=out6/k;end   
 im=sqrt(i1*i1+i2*i2+i3*i3+i4*i4+(i5*h5)^2+(i6*h6)^2);%
 time=time+T;  
 k=lim/im;
     if k>3
     k=3;end
 k11=k;k22=k;k33=k;k44=k;
     if flg5==1
     k55=k;end
     if flg6==1
     k66=k;end
  
 if time<1
     k11=0;k22=0;k33=0;k44=0;k55=0;k66=0;
 end
 if time>=1
     if time>=1.4
     low=1.02;end%1.02
     if time>=1.7
     low=0.512;end%0.512
 er6=u6*1.414-low;er5=u5*1.414-low;
%     if (er5<-0.06)||(er5>0.06)
%          if (er5<-0.06) 
%           if flg5==1
%           sum5=k;out5=k;end
%          flg5=0;end   
%     sum5=ki5*T*er5+sum5;out5=kp*er5+sum5;
%         if flg5==0 
%         k55=out5;end
%      if(out5>k)
%      flg5=1;out5=k;ki5=0;bao5=1;end
%      if(out5<0)
%      out5=0;ki5=0;bao5=1;end
%      if(bao5==0)
%      ki5=25;end
%      bao5=0;
%    end
%     if (er6<-0.06)||(er6>0.06)
%          if (er6<-0.06) 
%            if flg6==1
%            sum6=k;out6=k;end
%          flg6=0;end   
%      sum6=ki6*T*er6+sum6; out6=kp*er6+sum6;
%         if flg6==0 
%         k66=out6;end
%      if(out6>k)
%      flg6=1;out6=k;ki6=0;bao6=1;end
%      if(out6<0)
%      out6=0;ki6=0;bao6=1;end
%      if(bao6==0)
%      ki6=25;end
%      bao6=0;
%     end
 end
 
 k1=k11;k2=k22;k3=k33;k4=k44;k5=k55;k6=k66;k0=flg6;
end

== matlab function xieboduoji_13fangzhennow/node3/Subsystem1/RMS1/xunidiandao ==
  data: y1 output; u1 input; u2 input; u3 input; u4 input; u5 input; u6 input; y11 output; y2 output; y22 output; y3 output; y33 output; y4 output; y44 output; y5 output; y55 output; y6 output; y66 output; x output
function [y1,y11,y2,y22,y3,y33,y4,y44,y5,y55,y6,y66,x] = Algorithm(u1,u2,u3,u4,u5,u6)

%控制器参数
T=5e-5;
persistent time;
persistent sum1 sum2 sum3 sum4 sum5 sum6;
persistent sum11 sum22 sum33 sum44 sum55 sum66;
persistent a1 a11 a2 a22 a3 a33 a4 a44 a5 a55 a6 a66
dataType = 'double';

%首次赋值
 if isempty(time)
time=20e-5;
sum1=0;sum2=0;sum3=0;sum4=0;sum5=0;sum6=0;
sum11=0;sum22=0;sum33=0;sum44=0;sum55=0;sum66=0;
a1=0;a11=0;a2=0;a22=0;a3=0;a33=0;a4=0;a44=0;a5=0;a55=0;a6=0;a66=0;
 end

 time=time+T;
  
 if (time>=0.9)&&(time<1.0)
     sum1=sum1+u1;sum2=sum2+u2;sum3=sum3+u3;
     sum4=sum4+u4;sum5=sum5+u5;sum6=sum6+u6;
 end
 if time>=1.0
     a1=sum1*0.0005;a2=sum2*0.0005;a3=sum3*0.0005;
     a4=sum4*0.0005;a5=sum5*0.0005;a6=sum6*0.0005;
 end
  if (time>=1.9)&&(time<2.0)
     sum11=sum11+u1;sum22=sum22+u2;sum33=sum33+u3;
     sum44=sum44+u4;sum55=sum55+u5;sum66=sum66+u6;
 end
 if time>=2.0
     a11=sum11*0.0005;a22=sum22*0.0005;a33=sum33*0.0005;
     a44=sum44*0.0005;a55=sum55*0.0005;a66=sum66*0.0005;
 end
 y1=a1;y2=a2;y3=a3;y4=a4;y5=a5;y6=a6;
 y11=a11;y22=a22;y33=a33;y44=a44;y55=a55;y66=a66;x=time+sum1;
end

== matlab function xieboduoji_13fangzhennow/node3/谐波源/Subsystem1/RMS1/xunidiandao ==
  data: y1 output; u1 input; u2 input; u3 input; u4 input; u5 input; u6 input; y11 output; y2 output; y22 output; y3 output; y33 output; y4 output; y44 output; y5 output; y55 output; y6 output; y66 output; x output
function [y1,y11,y2,y22,y3,y33,y4,y44,y5,y55,y6,y66,x] = Algorithm(u1,u2,u3,u4,u5,u6)

%控制器参数
T=5e-5;
persistent time;
persistent sum1 sum2 sum3 sum4 sum5 sum6;
persistent sum11 sum22 sum33 sum44 sum55 sum66;
persistent a1 a11 a2 a22 a3 a33 a4 a44 a5 a55 a6 a66
dataType = 'double';

%首次赋值
 if isempty(time)
time=20e-5;
sum1=0;sum2=0;sum3=0;sum4=0;sum5=0;sum6=0;
sum11=0;sum22=0;sum33=0;sum44=0;sum55=0;sum66=0;
a1=0;a11=0;a2=0;a22=0;a3=0;a33=0;a4=0;a44=0;a5=0;a55=0;a6=0;a66=0;
 end

 time=time+T;
  
 if (time>=0.9)&&(time<1.0)
     sum1=sum1+u1;sum2=sum2+u2;sum3=sum3+u3;
     sum4=sum4+u4;sum5=sum5+u5;sum6=sum6+u6;
 end
 if time>=1.0
     a1=sum1*0.0005;a2=sum2*0.0005;a3=sum3*0.0005;
     a4=sum4*0.0005;a5=sum5*0.0005;a6=sum6*0.0005;
 end
  if (time>=1.9)&&(time<2.0)
     sum11=sum11+u1;sum22=sum22+u2;sum33=sum33+u3;
     sum44=sum44+u4;sum55=sum55+u5;sum66=sum66+u6;
 end
 if time>=2.0
     a11=sum11*0.0005;a22=sum22*0.0005;a33=sum33*0.0005;
     a44=sum44*0.0005;a55=sum55*0.0005;a66=sum66*0.0005;
 end
 y1=a1;y2=a2;y3=a3;y4=a4;y5=a5;y6=a6;
 y11=a11;y22=a22;y33=a33;y44=a44;y55=a55;y66=a66;x=time+sum1;
end

== matlab function xieboduoji_13fangzhennow/node3/PV15kW3/改进PLL1/PI/Embedded MATLAB Function ==
  data: Vgq input; w output
function w  = Algorithm(Vgq)

%控制器参数
T=5e-5;%控制周期

Kpllp=0.2;
Kplli=4;

persistent PLLsum;
persistent nsum2;

dataType = 'double';

%首次赋值
if isempty(PLLsum)
    PLLsum=0;
    nsum2=0;
end


w=Kpllp*Vgq+Kplli*(T*Vgq+PLLsum);
PLLsum=T*Vgq+PLLsum;
end

== matlab function xieboduoji_13fangzhennow/node3/谐波源/Subsystem2/RMS1/xunidiandao ==
  data: y1 output; u1 input; u2 input; u3 input; u4 input; u5 input; u6 input; y11 output; y2 output; y22 output; y3 output; y33 output; y4 output; y44 output; y5 output; y55 output; y6 output; y66 output; x output
function [y1,y11,y2,y22,y3,y33,y4,y44,y5,y55,y6,y66,x] = Algorithm(u1,u2,u3,u4,u5,u6)

%控制器参数
T=5e-5;
persistent time;
persistent sum1 sum2 sum3 sum4 sum5 sum6;
persistent sum11 sum22 sum33 sum44 sum55 sum66;
persistent a1 a11 a2 a22 a3 a33 a4 a44 a5 a55 a6 a66
dataType = 'double';

%首次赋值
 if isempty(time)
time=20e-5;
sum1=0;sum2=0;sum3=0;sum4=0;sum5=0;sum6=0;
sum11=0;sum22=0;sum33=0;sum44=0;sum55=0;sum66=0;
a1=0;a11=0;a2=0;a22=0;a3=0;a33=0;a4=0;a44=0;a5=0;a55=0;a6=0;a66=0;
 end

 time=time+T;
  
 if (time>=0.9)&&(time<1.0)
     sum1=sum1+u1;sum2=sum2+u2;sum3=sum3+u3;
     sum4=sum4+u4;sum5=sum5+u5;sum6=sum6+u6;
 end
 if time>=1.0
     a1=sum1*0.0005;a2=sum2*0.0005;a3=sum3*0.0005;
     a4=sum4*0.0005;a5=sum5*0.0005;a6=sum6*0.0005;
 end
  if (time>=1.9)&&(time<2.0)
     sum11=sum11+u1;sum22=sum22+u2;sum33=sum33+u3;
     sum44=sum44+u4;sum55=sum55+u5;sum66=sum66+u6;
 end
 if time>=2.0
     a11=sum11*0.0005;a22=sum22*0.0005;a33=sum33*0.0005;
     a44=sum44*0.0005;a55=sum55*0.0005;a66=sum66*0.0005;
 end
 y1=a1;y2=a2;y3=a3;y4=a4;y5=a5;y6=a6;
 y11=a11;y22=a22;y33=a33;y44=a44;y55=a55;y66=a66;x=time+sum1;
end

== matlab function xieboduoji_13fangzhennow/node4/Subsystem1/RMS1/xunidiandao ==
  data: y1 output; u1 input; u2 input; u3 input; u4 input; u5 input; u6 input; y11 output; y2 output; y22 output; y3 output; y33 output; y4 output; y44 output; y5 output; y55 output; y6 output; y66 output; x output
function [y1,y11,y2,y22,y3,y33,y4,y44,y5,y55,y6,y66,x] = Algorithm(u1,u2,u3,u4,u5,u6)

%控制器参数
T=5e-5;
persistent time;
persistent sum1 sum2 sum3 sum4 sum5 sum6;
persistent sum11 sum22 sum33 sum44 sum55 sum66;
persistent a1 a11 a2 a22 a3 a33 a4 a44 a5 a55 a6 a66
dataType = 'double';

%首次赋值
 if isempty(time)
time=20e-5;
sum1=0;sum2=0;sum3=0;sum4=0;sum5=0;sum6=0;
sum11=0;sum22=0;sum33=0;sum44=0;sum55=0;sum66=0;
a1=0;a11=0;a2=0;a22=0;a3=0;a33=0;a4=0;a44=0;a5=0;a55=0;a6=0;a66=0;
 end

 time=time+T;
  
 if (time>=0.9)&&(time<1.0)
     sum1=sum1+u1;sum2=sum2+u2;sum3=sum3+u3;
     sum4=sum4+u4;sum5=sum5+u5;sum6=sum6+u6;
 end
 if time>=1.0
     a1=sum1*0.0005;a2=sum2*0.0005;a3=sum3*0.0005;
     a4=sum4*0.0005;a5=sum5*0.0005;a6=sum6*0.0005;
 end
  if (time>=1.9)&&(time<2.0)
     sum11=sum11+u1;sum22=sum22+u2;sum33=sum33+u3;
     sum44=sum44+u4;sum55=sum55+u5;sum66=sum66+u6;
 end
 if time>=2.0
     a11=sum11*0.0005;a22=sum22*0.0005;a33=sum33*0.0005;
     a44=sum44*0.0005;a55=sum55*0.0005;a66=sum66*0.0005;
 end
 y1=a1;y2=a2;y3=a3;y4=a4;y5=a5;y6=a6;
 y11=a11;y22=a22;y33=a33;y44=a44;y55=a55;y66=a66;x=time+sum1;
end

== matlab function xieboduoji_13fangzhennow/node3/PV15kW3/谐波检测/Subsystem2/RMS1/xunidiandao ==
  data: k1 output; u1 input; i1 input; u2 input; i2 input; u3 input; i3 input; u4 input; i4 input; u5 input; i5 input; u6 input; k2 output; k3 output; k4 output; k5 output; k6 output; i6 input; k0 output
function [k1,k2,k3,k4,k5,k6,k0] = Algorithm(u1,i1,u2,i2,u3,i3,u4,i4,u5,i5,u6,i6)

%控制器参数
T=5e-5;
kp=0.01;
persistent low lim im k time;
persistent k11 k22 k33 k44 k55 k66;
persistent h6 flg6 sum6 out6 bao6 ki6;
persistent h5 flg5 sum5 out5 bao5 ki5;
dataType = 'double';

%首次赋值
 if isempty(k)
 low=1.244;lim=5;im=0;k=1;time=5e-5;%1.1
 k11=0;k22=0;k33=0;k44=0;k55=0;k66=0;
 h6=1;flg6=1;sum6=1;out6=1;bao6=0;ki6=25;
 h5=1;flg5=1;sum5=1;out5=1;bao5=0;ki5=25;
 end
%    if (flg5==0)&&(flg6==0)
%     if sqrt((i5*out5)^2+(i6*out6)^2)>lim
%          if (flg5>flg6)
%              flg5=1;
%          else
%              flg6=1;
%          end
%     end
%    end  
    if flg5==1
      h5=1;
    else h5=out5/k;end 
    if flg6==1
      h6=1;
    else h6=out6/k;end   
 im=sqrt(i1*i1+1*i2*i2+i3*i3+i4*i4+(i5*h5)^2+(i6*h6)^2);%
 time=time+T;  
 k=lim/im;
     if k>3
     k=3;end
 k11=k;k22=k;k33=k;k44=k;
     if flg5==1
     k55=k;end
     if flg6==1
     k66=k;end
  
 if time<1
     k11=0;k22=0;k33=0;k44=0;k55=0;k66=0;
 end
 if time>=1
     if time>=1.35
     low=1.02;end%1.02
     if time>=1.65
     low=0.7775;end%0.512
 er6=u6*1.414-low;er5=u5*1.414-low;
%     if (er5<-0.06)||(er5>0.06)
%          if (er5<-0.06) 
%           if flg5==1
%           sum5=k;out5=k;end
%          flg5=0;end   
%     sum5=ki5*T*er5+sum5;out5=kp*er5+sum5;
%         if flg5==0 
%         k55=out5;end
%      if(out5>k)
%      flg5=1;out5=k;ki5=0;bao5=1;end
%      if(out5<0)
%      out5=0;ki5=0;bao5=1;end
%      if(bao5==0)
%      ki5=25;end
%      bao5=0;
%    end
%     if (er6<-0.06)||(er6>0.06)
%          if (er6<-0.06) 
%            if flg6==1
%            sum6=k;out6=k;end
%          flg6=0;end   
%      sum6=ki6*T*er6+sum6; out6=kp*er6+sum6;
%         if flg6==0 
%         k66=out6;end
%      if(out6>k)
%      flg6=1;out6=k;ki6=0;bao6=1;end
%      if(out6<0)
%      out6=0;ki6=0;bao6=1;end
%      if(bao6==0)
%      ki6=25;end
%      bao6=0;
%     end
 end
 
 k1=k11;k2=k22;k3=k33;k4=k44;k5=k55;k6=k66;k0=flg6;
end

== matlab function xieboduoji_13fangzhennow/node4/Subsystem2/RMS1/xunidiandao ==
  data: y1 output; u1 input; u2 input; u3 input; u4 input; u5 input; u6 input; y11 output; y2 output; y22 output; y3 output; y33 output; y4 output; y44 output; y5 output; y55 output; y6 output; y66 output; x output
function [y1,y11,y2,y22,y3,y33,y4,y44,y5,y55,y6,y66,x] = Algorithm(u1,u2,u3,u4,u5,u6)

%控制器参数
T=5e-5;
persistent time;
persistent sum1 sum2 sum3 sum4 sum5 sum6;
persistent sum11 sum22 sum33 sum44 sum55 sum66;
persistent a1 a11 a2 a22 a3 a33 a4 a44 a5 a55 a6 a66
dataType = 'double';

%首次赋值
 if isempty(time)
time=20e-5;
sum1=0;sum2=0;sum3=0;sum4=0;sum5=0;sum6=0;
sum11=0;sum22=0;sum33=0;sum44=0;sum55=0;sum66=0;
a1=0;a11=0;a2=0;a22=0;a3=0;a33=0;a4=0;a44=0;a5=0;a55=0;a6=0;a66=0;
 end

 time=time+T;
  
 if (time>=0.9)&&(time<1.0)
     sum1=sum1+u1;sum2=sum2+u2;sum3=sum3+u3;
     sum4=sum4+u4;sum5=sum5+u5;sum6=sum6+u6;
 end
 if time>=1.0
     a1=sum1*0.0005;a2=sum2*0.0005;a3=sum3*0.0005;
     a4=sum4*0.0005;a5=sum5*0.0005;a6=sum6*0.0005;
 end
  if (time>=1.9)&&(time<2.0)
     sum11=sum11+u1;sum22=sum22+u2;sum33=sum33+u3;
     sum44=sum44+u4;sum55=sum55+u5;sum66=sum66+u6;
 end
 if time>=2.0
     a11=sum11*0.0005;a22=sum22*0.0005;a33=sum33*0.0005;
     a44=sum44*0.0005;a55=sum55*0.0005;a66=sum66*0.0005;
 end
 y1=a1;y2=a2;y3=a3;y4=a4;y5=a5;y6=a6;
 y11=a11;y22=a22;y33=a33;y44=a44;y55=a55;y66=a66;x=time+sum1;
end

== matlab function xieboduoji_13fangzhennow/node4/谐波源/Subsystem1/RMS1/xunidiandao ==
  data: y1 output; u1 input; u2 input; u3 input; u4 input; u5 input; u6 input; y11 output; y2 output; y22 output; y3 output; y33 output; y4 output; y44 output; y5 output; y55 output; y6 output; y66 output; x output
function [y1,y11,y2,y22,y3,y33,y4,y44,y5,y55,y6,y66,x] = Algorithm(u1,u2,u3,u4,u5,u6)

%控制器参数
T=5e-5;
persistent time;
persistent sum1 sum2 sum3 sum4 sum5 sum6;
persistent sum11 sum22 sum33 sum44 sum55 sum66;
persistent a1 a11 a2 a22 a3 a33 a4 a44 a5 a55 a6 a66
dataType = 'double';

%首次赋值
 if isempty(time)
time=20e-5;
sum1=0;sum2=0;sum3=0;sum4=0;sum5=0;sum6=0;
sum11=0;sum22=0;sum33=0;sum44=0;sum55=0;sum66=0;
a1=0;a11=0;a2=0;a22=0;a3=0;a33=0;a4=0;a44=0;a5=0;a55=0;a6=0;a66=0;
 end

 time=time+T;
  
 if (time>=0.9)&&(time<1.0)
     sum1=sum1+u1;sum2=sum2+u2;sum3=sum3+u3;
     sum4=sum4+u4;sum5=sum5+u5;sum6=sum6+u6;
 end
 if time>=1.0
     a1=sum1*0.0005;a2=sum2*0.0005;a3=sum3*0.0005;
     a4=sum4*0.0005;a5=sum5*0.0005;a6=sum6*0.0005;
 end
  if (time>=1.9)&&(time<2.0)
     sum11=sum11+u1;sum22=sum22+u2;sum33=sum33+u3;
     sum44=sum44+u4;sum55=sum55+u5;sum66=sum66+u6;
 end
 if time>=2.0
     a11=sum11*0.0005;a22=sum22*0.0005;a33=sum33*0.0005;
     a44=sum44*0.0005;a55=sum55*0.0005;a66=sum66*0.0005;
 end
 y1=a1;y2=a2;y3=a3;y4=a4;y5=a5;y6=a6;
 y11=a11;y22=a22;y33=a33;y44=a44;y55=a55;y66=a66;x=time+sum1;
end

== matlab function xieboduoji_13fangzhennow/node4/谐波源/Subsystem2/RMS1/xunidiandao ==
  data: y1 output; u1 input; u2 input; u3 input; u4 input; u5 input; u6 input; y11 output; y2 output; y22 output; y3 output; y33 output; y4 output; y44 output; y5 output; y55 output; y6 output; y66 output; x output
function [y1,y11,y2,y22,y3,y33,y4,y44,y5,y55,y6,y66,x] = Algorithm(u1,u2,u3,u4,u5,u6)

%控制器参数
T=5e-5;
persistent time;
persistent sum1 sum2 sum3 sum4 sum5 sum6;
persistent sum11 sum22 sum33 sum44 sum55 sum66;
persistent a1 a11 a2 a22 a3 a33 a4 a44 a5 a55 a6 a66
dataType = 'double';

%首次赋值
 if isempty(time)
time=20e-5;
sum1=0;sum2=0;sum3=0;sum4=0;sum5=0;sum6=0;
sum11=0;sum22=0;sum33=0;sum44=0;sum55=0;sum66=0;
a1=0;a11=0;a2=0;a22=0;a3=0;a33=0;a4=0;a44=0;a5=0;a55=0;a6=0;a66=0;
 end

 time=time+T;
  
 if (time>=0.9)&&(time<1.0)
     sum1=sum1+u1;sum2=sum2+u2;sum3=sum3+u3;
     sum4=sum4+u4;sum5=sum5+u5;sum6=sum6+u6;
 end
 if time>=1.0
     a1=sum1*0.0005;a2=sum2*0.0005;a3=sum3*0.0005;
     a4=sum4*0.0005;a5=sum5*0.0005;a6=sum6*0.0005;
 end
  if (time>=1.9)&&(time<2.0)
     sum11=sum11+u1;sum22=sum22+u2;sum33=sum33+u3;
     sum44=sum44+u4;sum55=sum55+u5;sum66=sum66+u6;
 end
 if time>=2.0
     a11=sum11*0.0005;a22=sum22*0.0005;a33=sum33*0.0005;
     a44=sum44*0.0005;a55=sum55*0.0005;a66=sum66*0.0005;
 end
 y1=a1;y2=a2;y3=a3;y4=a4;y5=a5;y6=a6;
 y11=a11;y22=a22;y33=a33;y44=a44;y55=a55;y66=a66;x=time+sum1;
end

== matlab function xieboduoji_13fangzhennow/node5/Subsystem1/RMS1/xunidiandao ==
  data: y1 output; u1 input; u2 input; u3 input; u4 input; u5 input; u6 input; y11 output; y2 output; y22 output; y3 output; y33 output; y4 output; y44 output; y5 output; y55 output; y6 output; y66 output; x output
function [y1,y11,y2,y22,y3,y33,y4,y44,y5,y55,y6,y66,x] = Algorithm(u1,u2,u3,u4,u5,u6)

%控制器参数
T=5e-5;
persistent time;
persistent sum1 sum2 sum3 sum4 sum5 sum6;
persistent sum11 sum22 sum33 sum44 sum55 sum66;
persistent a1 a11 a2 a22 a3 a33 a4 a44 a5 a55 a6 a66
dataType = 'double';

%首次赋值
 if isempty(time)
time=20e-5;
sum1=0;sum2=0;sum3=0;sum4=0;sum5=0;sum6=0;
sum11=0;sum22=0;sum33=0;sum44=0;sum55=0;sum66=0;
a1=0;a11=0;a2=0;a22=0;a3=0;a33=0;a4=0;a44=0;a5=0;a55=0;a6=0;a66=0;
 end

 time=time+T;
  
 if (time>=0.9)&&(time<1.0)
     sum1=sum1+u1;sum2=sum2+u2;sum3=sum3+u3;
     sum4=sum4+u4;sum5=sum5+u5;sum6=sum6+u6;
 end
 if time>=1.0
     a1=sum1*0.0005;a2=sum2*0.0005;a3=sum3*0.0005;
     a4=sum4*0.0005;a5=sum5*0.0005;a6=sum6*0.0005;
 end
  if (time>=1.9)&&(time<2.0)
     sum11=sum11+u1;sum22=sum22+u2;sum33=sum33+u3;
     sum44=sum44+u4;sum55=sum55+u5;sum66=sum66+u6;
 end
 if time>=2.0
     a11=sum11*0.0005;a22=sum22*0.0005;a33=sum33*0.0005;
     a44=sum44*0.0005;a55=sum55*0.0005;a66=sum66*0.0005;
 end
 y1=a1;y2=a2;y3=a3;y4=a4;y5=a5;y6=a6;
 y11=a11;y22=a22;y33=a33;y44=a44;y55=a55;y66=a66;x=time+sum1;
end

== matlab function xieboduoji_13fangzhennow/node3/PV15kW2/改进PLL1/PI/Embedded MATLAB Function ==
  data: Vgq input; w output
function w  = Algorithm(Vgq)

%控制器参数
T=5e-5;%控制周期

Kpllp=0.2;
Kplli=4;

persistent PLLsum;
persistent nsum2;

dataType = 'double';

%首次赋值
if isempty(PLLsum)
    PLLsum=0;
    nsum2=0;
end


w=Kpllp*Vgq+Kplli*(T*Vgq+PLLsum);
PLLsum=T*Vgq+PLLsum;
end
